simulink model "Lab2"  (R2021a)
settings: Solver=FixedStepAuto  StartTime=0.0  StopTime=5  FixedStep=0.001  RelTol=1e-3
values from neighbouring files (symbols this model uses):
  ci = 10    [initializare_model.m]
  EdR = 49584/8.32    (= 5959.61538462)    [initializare_model.m]
  k0 = 34930800    [initializare_model.m]
  Ti = 38+273    (= 311)    [initializare_model.m]
  V = 10    [initializare_model.m]
libraries: pid_lib x1
settings Model: Creator=Automatica  LastModifiedBy=Automatica

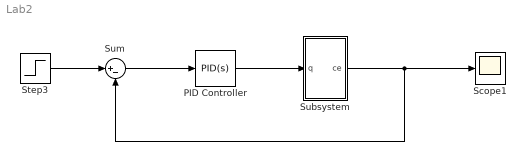
== system Lab2 ==
  PID Controller : pid_lib/PID Controller  Controller=PID  Form=Parallel  TimeDomain=Continuous-time  UseExternalTs=off  SampleTime=-1  IntegratorMethod=Forward Euler  FilterMethod=Forward Euler  ControllerParametersSource=internal  P=36  I=0.863  D=0  UseFilter=on  N=100  TunerSelectOption=Transfer Function Based (PID Tuner App)  InitialConditionSource=internal  InitialConditionForIntegrator=q  InitialConditionForFilter=0  DifferentiatorICPrevScaledInput=0  ExternalReset=none  TrackingMode=off  Kt=1  LimitOutput=off  SatLimitsSource=internal  UpperSaturationLimit=inf  LowerSaturationLimit=-inf  LinearizeAsGain=on  AntiWindupMode=none  Kb=1  POutMin=[]  POutMax=[]  IOutMin=[]  IOutMax=[]  DOutMin=[]  DOutMax=[]  NOutMin=[]  NOutMax=[]  SumOutMin=[]  SumOutMax=[]  SaturationOutMin=[]  SaturationOutMax=[]  PParamMin=[]  PParamMax=[]  IParamMin=[]  IParamMax=[]  DParamMin=[]  DParamMax=[]  NParamMin=[]  NParamMax=[]  KbParamMin=[]  KbParamMax=[]  KtParamMin=[]  KtParamMax=[]  KbOutMin=[]  KbOutMax=[]  KtOutMin=[]  KtOutMax=[]  IntegratorOutMin=[]  IntegratorOutMax=[]  FilterOutMin=[]  FilterOutMax=[]  SumI1OutMin=[]  SumI1OutMax=[]  SumI2OutMin=[]  SumI2OutMax=[]  SumI3OutMin=[]  SumI3OutMax=[]  SumI4OutMin=[]  SumI4OutMax=[]  SumDOutMin=[]  SumDOutMax=[]  DifferentiatorOutMin=[]  DifferentiatorOutMax=[]  FilterDiffOutCoefMin=[]  FilterDiffOutCoefMax=[]  ReciprocalOutMin=[]  ReciprocalOutMax=[]  SumDenOutMin=[]  SumDenOutMax=[]  SumNumOutMin=[]  SumNumOutMax=[]  DivideOutMin=[]  DivideOutMax=[]  UdiffTsProdOutMin=[]  UdiffTsProdOutMax=[]  NTsProdOutMin=[]  NTsProdOutMax=[]  UintegralTsProdOutMin=[]  UintegralTsProdOutMax=[]  UngainTsProdOutMin=[]  UngainTsProdOutMax=[]  IntegratorContinuousStateAttributes=''  IntegratorStateMustResolveToSignalObject=off  IntegratorRTWStateStorageClass=Auto  FilterContinuousStateAttributes=''  FilterStateMustResolveToSignalObject=off  FilterRTWStateStorageClass=Auto  ParallelPVariant=InternalParameters  IdealPVariant=Disabled  IVariant=InternalParameters  DVariant=InternalParameters  IntegratorVariant=Continuous  SatVariant=Disabled  AWVariant=Passthrough  PCopyVariant=Disabled  TRVariant=Disabled  FdbkBlocksVariant=Forward  IdealPFdbkVariant=Disabled  SatFdbkVariant=Disabled  DerivativeFilterVariant=ContFilter  NVariant=InternalParameters  NCopyVariant=Disabled  FilterICVariant=InternalICsFilter  IntegratorICVariant=InternalICs  ExternalResetVariant=Disabled  TRSumVariant=Passthrough  SumFdbkVariant=Disabled  SumVariant=Sum_PID  TsampFilterVariant=InternalTs  TsampNgainVariant=Passthrough  TsampIntegralVariant=Passthrough  ExternalSaturationOutDataTypeStr=Inherit: Same as second input
  Scope1 : Scope
  Step3 : Step  Time=0  Before=8.574  After=8.674  SampleTime=0
  Subsystem : Subsystem
  Sum : Sum  Inputs=|+-
  wires:
  Step3/1 -> Sum/1
  Sum/1 -> PID Controller/1
  PID Controller/1 -> Subsystem/1(q)
  Subsystem/1(ce) -> Scope1/1, Sum/2

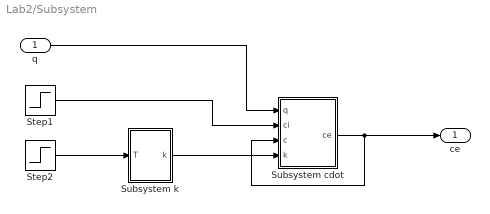
== system Lab2/Subsystem ==
  q : Inport
  Step1 : Step  Time=0  Before=ci  After=ci  SampleTime=0
  Step2 : Step  Before=Ti  After=Ti  SampleTime=0
  Subsystem cdot : Subsystem
  Subsystem k : Subsystem
  ce : Outport
  wires:
  Subsystem cdot/1(ce) -> ce/1, Subsystem cdot/3(c)
  Subsystem k/1(k) -> Subsystem cdot/4(k)
  Step2/1 -> Subsystem k/1(T)
  Step1/1 -> Subsystem cdot/2(ci)
  q/1 -> Subsystem cdot/1(q)

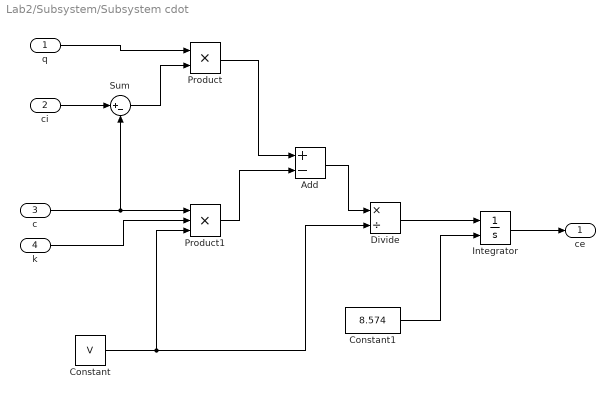
== system Lab2/Subsystem/Subsystem cdot ==
  q : Inport
  ci : Inport  Port=2
  c : Inport  Port=3
  k : Inport  Port=4
  Add : Sum  Inputs=+-
  Constant : Constant  Value=V
  Constant1 : Constant  Value=8.574
  Divide : Product  Inputs=*/
  Integrator : Integrator  InitialConditionSource=external
  Product : Product
  Product1 : Product  Inputs=3
  Sum : Sum  Inputs=|+-
  ce : Outport
  wires:
  ci/1 -> Sum/1
  Sum/1 -> Product/2
  q/1 -> Product/1
  Product/1 -> Add/1
  Product1/1 -> Add/2
  c/1 -> Sum/2, Product1/1
  k/1 -> Product1/2
  Constant/1 -> Product1/3, Divide/2
  Add/1 -> Divide/1
  Divide/1 -> Integrator/1
  Integrator/1 -> ce/1
  Constant1/1 -> Integrator/2

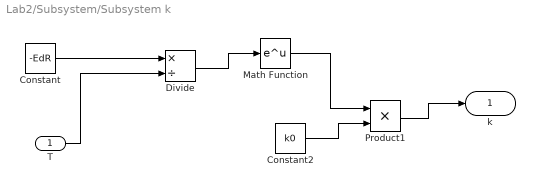
== system Lab2/Subsystem/Subsystem k ==
  T : Inport
  Constant : Constant  Value=-EdR
  Constant2 : Constant  Value=k0
  Divide : Product  Inputs=*/
  Math Function : Math  SaturateOnIntegerOverflow=on
  Product1 : Product
  k : Outport
  wires:
  Constant/1 -> Divide/1
  T/1 -> Divide/2
  Constant2/1 -> Product1/2
  Product1/1 -> k/1
  Math Function/1 -> Product1/1
  Divide/1 -> Math Function/1
